simulink model "HW3_1c"  (Simulink 8.9)
settings: Solver=ode45  StartTime=0.0  StopTime=10.0  RelTol=1e-3  EnableMultiTasking=on
undefined symbols (not defined in the file): sigbuilder_block
settings Model: Creator=Gopanraj  LastModifiedBy=Soutrik
settings OptimizationCC: ExpressionDepthLimit=2147483647
settings DebuggingCC: SolverPrmCheckMsg=warning
settings GRTTargetCC: CombineOutputUpdateFcns=on  GRTInterface=off

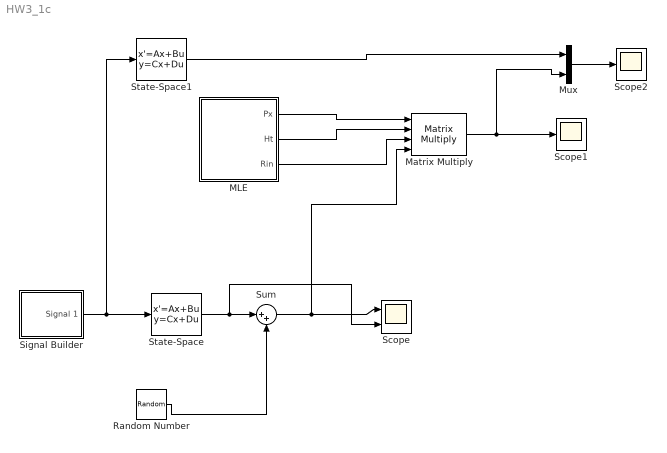
== system HW3_1c ==
  MLE : MATLAB Function  TreatAsAtomicUnit=on
  Matrix Multiply : Product  Inputs=4  Multiplication=Matrix(*)
  Mux : Mux  Inputs=2
  Random Number : RandomNumber  Variance=[0.0001, 0.0000001, 0.00002, 0.00002]  SampleTime=0.01
  Scope : Scope  NumInputPorts=2
  Scope1 : Scope
  Scope2 : Scope
  Signal Builder : Subsystem  Tag=STV Subsys  LoadFcn=sigbuilder_block('load');  StartFcn=sigbuilder_block('start');  StopFcn=sigbuilder_block('stop');  ClipboardFcn=sigbuilder_block('clipboard');  mask(Sigbuilder block){tuvar=[0:10]}
      mask help: Simulink:masks:SigbuilderBlock_MD
      mask init:
      | if ~strcmp(get_param(bdroot(gcbh),'SimulationStatus'),'stopped') tuvar = sigbuilder_block('maskInit'); end
      settings: CopyFcn=sigbuilder_block('copy');  DeleteFcn=sigbuilder_block('delete');  ModelCloseFcn=sigbuilder_block('modelClose');  PreSaveFcn=sigbuilder_block('preSave');  PauseFcn=sigbuilder_block('pause');  ContinueFcn=sigbuilder_block('continue');  NameChangeFcn=sigbuilder_block('namechange');  OpenFcn=sigbuilder_block('open',[6 21 1012.5 492 ]);  CloseFcn=sigbuilder_block('close');
      mask Display: plot(0, 0, 100, 100,[2, 2, 32, 32, 2], [68, 8, 8, 68, 68],[32, 2], [38, 38], [32, 19, 2],[53, 60, 44], [32, 17, 17, 2],[16, 16, 31, 31]);txt = getActiveGroup(gcbh);text(2, 100, txt,'verticalAlignment', 'top');
  State-Space : StateSpace  A=|  B=|  C=|  D=[0 ;0; 0 ;0]  X0=0  ContinuousStateAttributes={ 'Pitch_angle', 'Pitch_rate' ,'X_Axis_Velocity', 'Z_Axis_Velocity'}
      A=|
      | [0 1.0000 0 0;
      | 0 -0.9965 0 -0.3000;
      | -0.3197 -0.5176 -0.0100 -0.7000;
      | 0 0 -0.0005 -0.9924]
      B=|
      | [ 0;
      | -0.0013;
      | 0.0001;
      | -0.0201];
      C=|
      | [0 0 0.9963 0.0862;
      | 0 0 -0.0001 0.0017;
      | 1.0000 0 0 0;
      | 0 1.0000 0 0]
  State-Space1 : StateSpace  A=|  B=|  C=[ 1 0 0 0; 0 1 0 0; 0 0 1 0; 0 0 0 1];  D=[0 ;0; 0 ;0]  X0=0  ContinuousStateAttributes={ 'Pitch_angle', 'Pitch_rate' ,'X_Axis_Velocity', 'Z_Axis_Velocity'}
      A=|
      | [0 1.0000 0 0;
      | 0 -0.9965 0 -0.3000;
      | -0.3197 -0.5176 -0.0100 -0.7000;
      | 0 0 -0.0005 -0.9924]
      B=|
      | [ 0;
      | -0.0013;
      | 0.0001;
      | -0.0201];
  Sum : Sum  Inputs=|++
  wires:
  Signal Builder/1(Signal 1) -> State-Space/1, State-Space1/1
  Random Number/1 -> Sum/2
  Sum/1 -> Scope/1, Matrix Multiply/4
  State-Space/1 -> Scope/2, Sum/1
  MLE/1(Px) -> Matrix Multiply/1
  MLE/2(Ht) -> Matrix Multiply/2
  MLE/3(Rin) -> Matrix Multiply/3
  Matrix Multiply/1 -> Scope1/1, Mux/2
  State-Space1/1 -> Mux/1
  Mux/1 -> Scope2/1

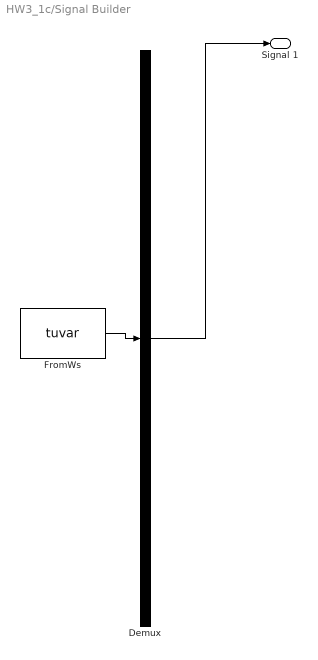
== system HW3_1c/Signal Builder ==
  Demux : Demux  Tag=STV Demux  Outputs=1
  FromWs : FromWorkspace  Tag=STV FromWs  VariableName=tuvar  SampleTime=0  SigBuilderData=DataTag0  VnvData=DataTag1
      SigBuilderData=|
      | common.afterFinalStr = 'Extrapolate'
      | common.sampleTime = 0
      | dataSet.timeRange = [0 10]
      | dataSet.name = 'Group 1'
      | sbobj.Groups.Name = 'Group 1'
      | sbobj.Groups.Signals.Name = 'Signal 1'
      | sbobj.Groups.Signals.XData = [0 1 1 2 2 3 3 10]
      | sbobj.Groups.Signals.YData = [0 0 50 50 -50 -50 0 0]
  Signal 1 : Outport  Tag=STV Outport
  wires:
  Demux/1 -> Signal 1/1
  FromWs/1 -> Demux/1

== matlab function MLE ==
  data: Px output double; Ht output double; Rin output double
function [Px,Ht,Rin] = fcn
a =[0 1.0000 0 0;
0 -0.9965 0 -0.3000;
-0.3197 -0.5176 -0.0100 -0.7000;
0 0 -0.0005 -0.9924];


c =[0 0 0.9963 0.0862;
0 0 -0.0001 0.0017;
1.0000 0 0 0;
0 1.0000 0 0];

cov=[0.0001, 0.0000001, 0.00002, 0.00002];

R=diag(cov);
Rin=inv(R);
H=c;
Ht=H';
Px=inv(Ht*Rin*H);
